simulink model "sys_model"  (R2020b)
settings: Solver=VariableStepAuto  StartTime=0.0  StopTime=2  RelTol=1e-3
values from neighbouring files (symbols this model uses):
  b = 3.5077E-6    [sys_dict.sldd]
  J = 3.2284E-6    [sys_dict.sldd]
  K = 0.0274    [sys_dict.sldd]
  Kd = 350.0    [sys_dict.sldd]
  Ki = 250.0    [sys_dict.sldd]
  Kp = 100.0    [sys_dict.sldd]
  L = 2.75E-6    [sys_dict.sldd]
  R = 4.0    [sys_dict.sldd]
  Ts = 0.01    [sys_dict.sldd]
settings Model: DataDictionary=sys_dict.sldd  Creator=Rasika Shejul  LastModifiedBy=Rushikesh

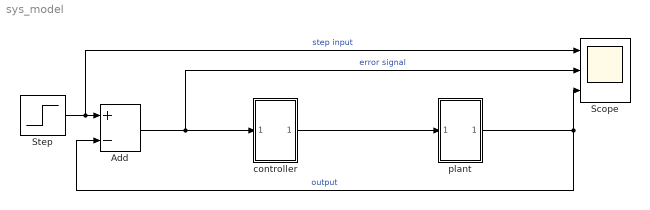
== system sys_model ==
  Add : Sum  Inputs=+-
  Scope : Scope  NumInputPorts=3
  Step : Step  SampleTime=0
  controller : Subsystem
  plant : Subsystem
  wires:
  Add/1 -> Scope/2, controller/1(In1)  "error signal"
  plant/1(theta) -> Add/2, Scope/3  "output"
  Step/1 -> Scope/1, Add/1  "step input"
  controller/1(Out1) -> plant/1(In1)

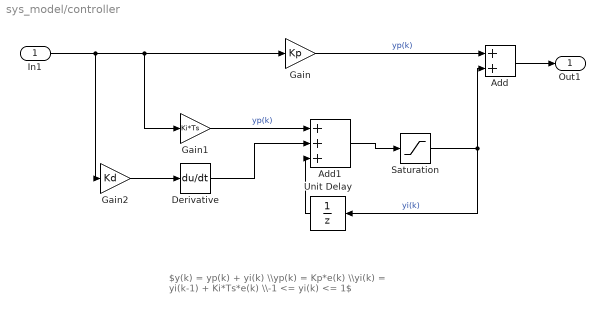
== system sys_model/controller ==
  note: $y(k) = yp(k) + yi(k) \\yp(k) = Kp*e(k) \\yi(k) = yi(k-1) + Ki*Ts*e(k) \\-1 <= yi(k) <= 1$
  In1 : Inport
  Add : Sum
  Add1 : Sum  Inputs=+++
  Derivative : Derivative
  Gain : Gain  Gain=Kp
  Gain1 : Gain  Gain=Ki*Ts
  Gain2 : Gain  Gain=Kd
  Saturation : Saturate  UpperLimit=1  LowerLimit=-1
  Unit Delay : UnitDelay  SampleTime=-1  HasFrameUpgradeWarning=on
  Out1 : Outport
  wires:
  Gain1/1 -> Add1/1  "yp(k)"
  Add/1 -> Out1/1
  Unit Delay/1 -> Add1/3
  Gain/1 -> Add/1  "yp(k)"
  In1/1 -> Gain2/1, Gain1/1, Gain/1
  Saturation/1 -> Add/2, Unit Delay/1  "yi(k)"
  Add1/1 -> Saturation/1
  Derivative/1 -> Add1/2
  Gain2/1 -> Derivative/1

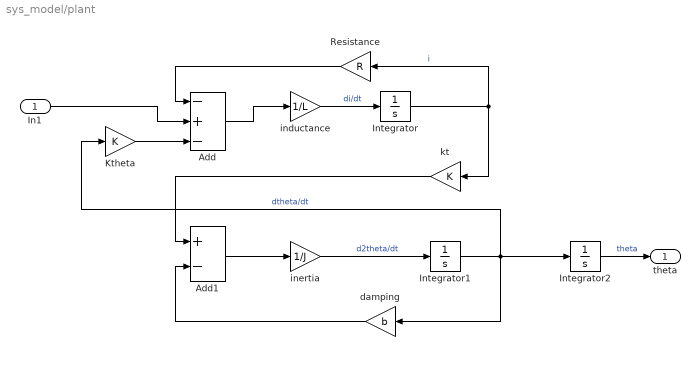
== system sys_model/plant ==
  In1 : Inport
  Add : Sum  Inputs=-+-
  Add1 : Sum  Inputs=+-
  Integrator : Integrator
  Integrator1 : Integrator
  Integrator2 : Integrator
  Ktheta : Gain  Gain=K
  Resistance : Gain  Gain=R
  damping : Gain  Gain=b
  inductance : Gain  Gain=1/L
  inertia : Gain  Gain=1/J
  kt : Gain  Gain=K
  theta : Outport
  wires:
  Ktheta/1 -> Add/3
  Integrator1/1 -> Integrator2/1, damping/1, Ktheta/1  "dtheta/dt"
  Integrator/1 -> Resistance/1, kt/1  "i"
  damping/1 -> Add1/2
  Add1/1 -> inertia/1
  Resistance/1 -> Add/1
  kt/1 -> Add1/1
  inertia/1 -> Integrator1/1  "d2theta/dt"
  inductance/1 -> Integrator/1  "di/dt"
  Add/1 -> inductance/1
  In1/1 -> Add/2
  Integrator2/1 -> theta/1  "theta"
